simulink model "pidtune_sim"  (R2024a)
settings: Solver=VariableStepAuto  StartTime=0.0  StopTime=20  RelTol=1e-3
settings Model: Creator=hello.welcometothisdevice  LastModifiedBy=hello.welcometothisdevice
settings SolverCC: MaxConsecutiveMinStep=2

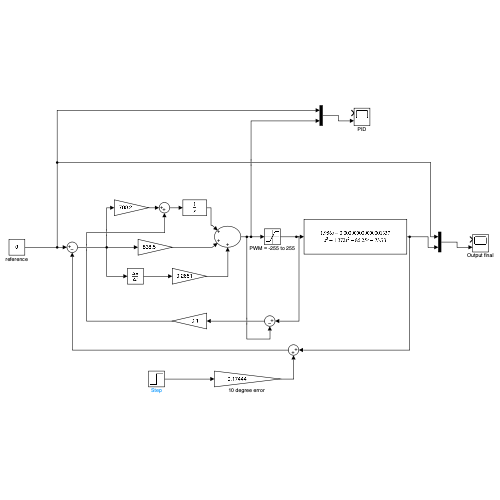
[thumbnail: Simulink's stored preview of the top-level diagram]
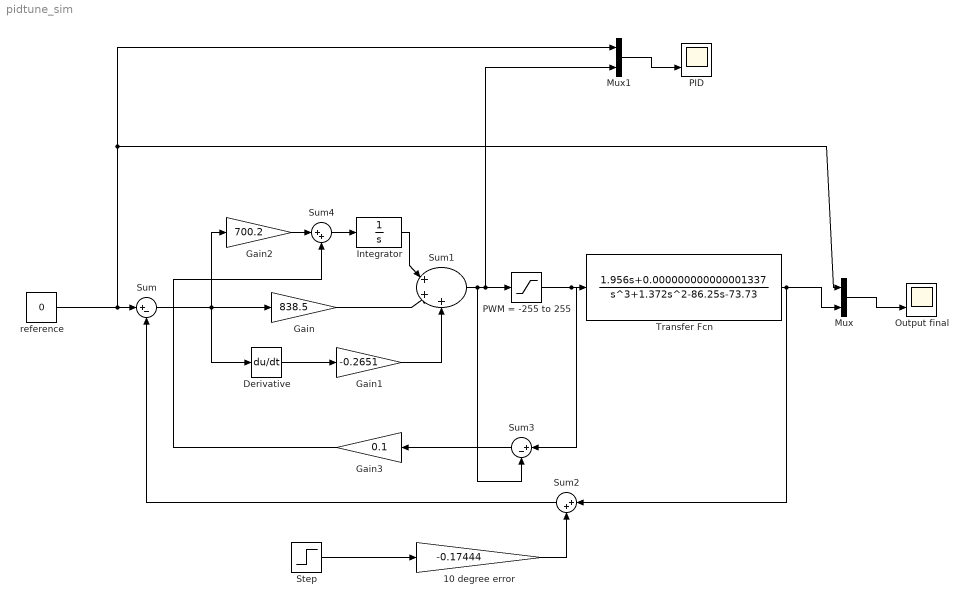
== system pidtune_sim ==
  "10 degree error " : Gain  Gain=-0.17444
  Derivative : Derivative
  Gain : Gain  Gain=838.5
  Gain1 : Gain  Gain=-0.2651
  Gain2 : Gain  Gain=700.2
  Gain3 : Gain  Gain=0.1
  Integrator : Integrator
  Mux : Mux  Inputs=2
  Mux1 : Mux  Inputs=2
  Output final : Scope  NumInputPorts=2
  PID : Scope  NumInputPorts=2
  PWM = -255 to 255 : Saturate  UpperLimit=255  LowerLimit=-255
  Step : Step  SampleTime=0
  Sum : Sum  Inputs=|+-
  Sum1 : Sum  Inputs=|+++
  Sum2 : Sum  Inputs=|++
  Sum3 : Sum  Inputs=|+-
  Sum4 : Sum  Inputs=|++
  Transfer Fcn : TransferFcn  Numerator=[1.956 0.000000000000001337]  Denominator=[1 1.372 -86.25 -73.73]  ParameterTunability=Optimized
  reference : Constant  Value=0
  wires:
  Transfer Fcn/1 -> Sum2/1, Mux/2
  reference/1 -> Mux1/1, Mux/1, Sum/1
  Sum1/1 -> Mux1/2, PWM = -255 to 255/1, Sum3/2
  Sum/1 -> Gain2/1, Derivative/1, Gain/1
  Gain/1 -> Sum1/2
  Gain1/1 -> Sum1/3
  Integrator/1 -> Sum1/1
  Derivative/1 -> Gain1/1
  Mux/1 -> Output final/2
  Mux1/1 -> PID/2
  Sum2/1 -> Sum/2
  "10 degree error "/1 -> Sum2/2
  PWM = -255 to 255/1 -> Sum3/1, Transfer Fcn/1
  Step/1 -> "10 degree error "/1
  Gain2/1 -> Sum4/1
  Sum4/1 -> Integrator/1
  Sum3/1 -> Gain3/1
  Gain3/1 -> Sum4/2
